simulink model "PIL_NO_RPI_new"  (R2021a)
settings: Solver=FixedStepAuto  StartTime=0.0  StopTime=60  FixedStep=0.001  RelTol=1e-3  EnableMultiTasking=on
values from neighbouring files (symbols this model uses):
  den_lpf_d = den_lpf20    [Mainframe_init.m]    (also in load_autopilot.m)
  Enable_Gyros = 0    [Mainframe_init.m]
  Enable_INS = 0    [Mainframe_init.m]
  num_lpf_d = num_lpf20    [Mainframe_init.m]    (also in load_autopilot.m)
undefined symbols (not defined in the file or in its folder): act_dmp, act_omega, Actuator, Aerodynamics, aMode, Autopilot, AUX, c_b_WGS, c_be, c_flat, c_grav, c_h_geop0, c_h_geope, c_pa0, c_pe, c_r0, c_rot, c_rsma, c_Tmp0, d_siB_0, d_siB_max, d_siB_min, dd_siB_max, dd_siB_min, dev, DiscIntNeverNeededParam, e_pa, e_Tmp, fin_maxrate, flag_I_act_switch, flag_I_aero_switch, flag_I_flat, flag_I_gravity_switch, flag_I_rot, h_bkpts_m, hcr, HIL_Data, JMMM_0, JMMM_e, JSPB_e, Ki_phi_vec, Kp_p_vec, Kp_phi_vec, lat_0, lon_0, Mass_Props, mB_0, mM_0, mM_e, National_Instruments, Newton, p, pBII_0, PCIe, phi, pMPB, pNPB, propellant_kg, prp_FBPB, prp_mdot ... (+40)
libraries: simulink x32, simulink_extras x23, aerolibcommonsys x4, pil_lib x2, custom_blocks x1, px4lib x1, sldrtlib x1, aerolibnav x1
(part 4 of 16)

== system PIL_NO_RPI_new/Non-linear Flight Dynamic Model1/GRM_Airframe/fin_actuators/Rudder3 ==
  siB_c : Inport
  tRRR : Inport  Port=2
  Add : Sum  Inputs=+-
  Add1 : Sum  Inputs=+-
  Add3 : Sum  Inputs=+++
  Constant1 : Constant  Value=Actuator.fin4_bias
      settings: AttributesFormatString=%<Value>
  Gain : Gain  Gain=omega^2
  Gain2 : Gain  Gain=2*dmp*omega  Multiplication=Matrix(K*u)
  Gain3 : Gain  Gain=unc_bl
  Gain4 : Gain  Gain=Actuator.fin4_scale
      settings: AttributesFormatString=%<Gain>
  Integrator : Integrator  ExternalReset=either  InitialCondition=d_siB_0
  Integrator1 : Integrator  InitialCondition=siB_0  LimitOutput=on  UpperSaturationLimit=siB_max  LowerSaturationLimit=siB_min  ShowSaturationPort=on
  Limiting_Acceleration : MATLAB Function  TreatAsAtomicUnit=on
  Limiting_Rate : MATLAB Function  TreatAsAtomicUnit=on
  Saturation : Saturate  UpperLimit=siB_max  LowerLimit=siB_min
  Saturation1 : Saturate  UpperLimit=siB_max  LowerLimit=siB_min
  Sign : Signum
  siB : Outport  VectorParamsAs1DForOutWhenUnconnected=off
  d_siB : Outport  Port=2  VectorParamsAs1DForOutWhenUnconnected=off
  dd_siB : Outport  Port=3  VectorParamsAs1DForOutWhenUnconnected=off
  wires:
  Saturation1/1 -> siB/1, [siB]  "siB"
  Integrator1/2 -> Integrator/2  "sat"
  Gain3/1 -> Add3/3
  Sign/1 -> Gain3/1
  tRRR/1 -> Sign/1  "tRRR"
  Integrator1/1 -> Gain4/1, Add/2  "siB"
  Add1/1 -> Limiting_Acceleration/3(dd_siB)  "dd_siB"
  Gain2/1 -> Add1/2
  Gain/1 -> Add1/1
  Add/1 -> Gain/1
  Limiting_Acceleration/1(dd_siB_l) -> Integrator/1, dd_siB/1  "dd_siB_l"
  Limiting_Rate/1(d_siB_l) -> d_siB/1, [d_siB], Integrator1/1  "d_siB_l"
  Integrator/1 -> Limiting_Rate/2(d_siB), Gain2/1  "d_siB"
  Saturation/1 -> Add/1
  Add3/1 -> Saturation1/1
  siB_c/1 -> Saturation/1  "siB_c"
  [d_siB] -> Limiting_Acceleration/2(d_siB)
  [siB] -> Limiting_Acceleration/1(siB)
  [siB] -> Limiting_Rate/1(siB)
  Constant1/1 -> Add3/1
  Gain4/1 -> Add3/2

== system PIL_NO_RPI_new/Non-linear Flight Dynamic Model1/GRM_Airframe/fin_actuators/control_allocation ==
  siB : Inport
  d_siB : Inport  Port=2
  dd_siB : Inport  Port=3
  Constant8 : Constant  Value=Tr3r4
  Product : Product  Multiplication=Matrix(*)
  Product1 : Product  Multiplication=Matrix(*)
  Product2 : Product  Multiplication=Matrix(*)
  Tr3r4 : Outport  VectorParamsAs1DForOutWhenUnconnected=off
  finB : Outport  Port=2  VectorParamsAs1DForOutWhenUnconnected=off
  d_finB : Outport  Port=3  VectorParamsAs1DForOutWhenUnconnected=off
  dd_finB : Outport  Port=4  VectorParamsAs1DForOutWhenUnconnected=off
  wires:
  Product/1 -> finB/1  "afinB"
  Constant8/1 -> Tr3r4/1, Product2/1, Product1/1, Product/1  "Tr3r4"
  siB/1 -> Product/2
  d_siB/1 -> Product1/2
  Product1/1 -> d_finB/1  "d_afinB"
  dd_siB/1 -> Product2/2
  Product2/1 -> dd_finB/1  "dd_afinB"

== system PIL_NO_RPI_new/Non-linear Flight Dynamic Model1/GRM_Airframe/gravity/launch_rail ==
  gBG_c : Inport
  hBE : Inport  Port=2
  Constant1 : Constant  Value=flag_I_gravity_switch
  Constant3 : Constant  Value=0
  Subtract : Sum  Inputs=++-
  Switch : Switch  Criteria=u2 > Threshold  Threshold=0.05
  Vector Concatenate : Concatenate  NumInputs=3
  initial_altitude : Subsystem
  gBG : Outport  VectorParamsAs1DForOutWhenUnconnected=off
  wires:
  Constant1/1 -> Subtract/2
  hBE/1 -> Subtract/1
  Subtract/1 -> Switch/2
  Constant3/1 -> Vector Concatenate/1, Vector Concatenate/2, Vector Concatenate/3
  Switch/1 -> gBG/1  "gBG"
  Vector Concatenate/1 -> Switch/3
  gBG_c/1 -> Switch/1
  initial_altitude/1(hBE_0) -> Subtract/3

== system PIL_NO_RPI_new/Non-linear Flight Dynamic Model1/GRM_Airframe/motion_kinematics/calc_motion_kinematics ==
  lat : Inport
  lon : Inport  Port=2
  qIB : Inport  Port=3
  calc_transformation_matrix : Subsystem
  earth_rotation : Subsystem
  wIEE : Outport  VectorParamsAs1DForOutWhenUnconnected=off
  TIE : Outport  Port=2  VectorParamsAs1DForOutWhenUnconnected=off
  TEB : Outport  Port=3  VectorParamsAs1DForOutWhenUnconnected=off
  TGB : Outport  Port=4  VectorParamsAs1DForOutWhenUnconnected=off
  TEG : Outport  Port=5  VectorParamsAs1DForOutWhenUnconnected=off
  wEGG : Outport  Port=6  VectorParamsAs1DForOutWhenUnconnected=off
  TIB : Outport  Port=7  VectorParamsAs1DForOutWhenUnconnected=off
  wires:
  earth_rotation/1(wIEE) -> wIEE/1
  earth_rotation/2(TIE) -> TIE/1
  earth_rotation/5(TEG) -> TEG/1
  earth_rotation/6(wEGG) -> wEGG/1
  lon/1 -> earth_rotation/2(lon)
  lat/1 -> earth_rotation/1(lat)
  earth_rotation/3(qIE) -> calc_transformation_matrix/1(qIE)
  earth_rotation/4(qEG) -> calc_transformation_matrix/2(qEG)
  qIB/1 -> calc_transformation_matrix/3(qIB)
  calc_transformation_matrix/1(TEB) -> TEB/1
  calc_transformation_matrix/2(TGB) -> TGB/1
  calc_transformation_matrix/3(TIB) -> TIB/1

== system PIL_NO_RPI_new/Non-linear Flight Dynamic Model1/GRM_Airframe/propulsion/prp_look_up ==
  env_glbl_bus : Inport
  Bus Selector1 : BusSelector  OutputSignals=T_sim_glbl,T_sim_lnch
  Constant : Constant  Value=0
  Constant1 : Constant  Value=0
  Saturation : Saturate  UpperLimit=prp_T(end)  LowerLimit=0
      settings: AttributesFormatString=|
      | %<UpperLimit>
      | %<LowerLimit>
  Subtract : Sum  Inputs=+-
  Switch : Switch  Criteria=u2 > Threshold
  Switch1 : Switch  Criteria=u2 > Threshold
  Vector Concatenate : Concatenate  NumInputs=3
  thrust_lookup : Lookup_n-D  NumberOfTableDimensions=1  BreakpointsForDimension1=prp_T  Table=prp_FBPB  ExtrapMethod=Clip  UseLastTableValue=on  InternalRulePriority=Speed  RndMeth=Simplest  InputSameDT=on
  FBPM : Outport  VectorParamsAs1DForOutWhenUnconnected=off
  wires:
  Bus Selector1/2 -> Subtract/2  "<T_sim_lnch>"
  Switch/1 -> Saturation/1, Switch1/2, Switch1/3
  thrust_lookup/1 -> Switch1/1
  Bus Selector1/1 -> Subtract/1  "<T_sim_glbl>"
  env_glbl_bus/1 -> Bus Selector1/1
  Constant/1 -> Switch/3
  Subtract/1 -> Switch/1, Switch/2
  Saturation/1 -> thrust_lookup/1
  Vector Concatenate/1 -> FBPM/1  "FBPM"
  Constant1/1 -> Vector Concatenate/3, Vector Concatenate/2
  Switch1/1 -> Vector Concatenate/1  "a_FBPM"

== system PIL_NO_RPI_new/Non-linear Flight Dynamic Model1/GRM_Airframe/propulsion/prp_uncertainty ==
  FBPM : Inport
  wab : Inport  Port=2
  3_rot_mat : Subsystem  mask(Rotation um 1, 2 oder 3 Achsen){rot_1=Rotation um z-Achse, rot_2=Rotation um y-Achse, rot_3=Rotation um x-Achse}
      mask prompts: rot_1 "1. Rotation"; rot_2 "2. Rotation"; rot_3 "3. Rotation"
      mask help:
      | Dieser Block liefert die Rotationsmatrix T12 für den Fall zurück, dass sich das Ziel-Koordinatensystem (1) durch Drehungen um 1, 2 oder 3 Achsen gegenüber dem Ausgangskoordinatensystem (2) beschreiben lässt (passive Drehung).
      |
      | Die Anzahl der Rotation sowie die Reihenfolge ist frei einstellbar.
      |
      | Die Rotationswinkel haben die Einheit [rad].
      mask TypeOptions rot_1: Rotation um x-Achse | Rotation um y-Achse | Rotation um z-Achse
      mask TypeOptions rot_2: Rotation um x-Achse | Rotation um y-Achse | Rotation um z-Achse
      mask TypeOptions rot_3: Rotation um x-Achse | Rotation um y-Achse | Rotation um z-Achse
  Bus Selector : BusSelector  OutputSignals=pBPB
  Product : Product  Multiplication=Matrix(*)
  Product1 : Product
  Subtract : Sum  Inputs=+-
  Thrust_rot_z : Constant  Value=unc_prp_z
  cross_product : Subsystem
      mask help: cross product r3 = r1 x r2
      mask Help:
      | Name:
      | 
      |     cross_product
      | 
      | Description:
      | 
      |     This block implements the cross product r3 = r1 x r2.
      | 
      | Inputs  [size] [data type] [unit]:
      | 
      |     vector 1  [3] [double] [-]
      |     vector 2  [3] [double] [-]
      | 
      | Outputs  [size] [data type] [unit]:
      | 
      |     resulting vector  [3] [double] [-]
      mask Display: disp(' r3 = r1 x r2')
  pNPB : Constant  Value=pNPB
  thrust_rot_x : Constant  Value=unc_prp_x
  thrust_rot_y : Constant  Value=unc_prp_y
  uncert_thrust : Constant  Value=unc_prp_scale
  FBPB : Outport  VectorParamsAs1DForOutWhenUnconnected=off
  MBPB : Outport  Port=2  VectorParamsAs1DForOutWhenUnconnected=off
  wires:
  Thrust_rot_z/1 -> 3_rot_mat/1(wi1)
  thrust_rot_x/1 -> 3_rot_mat/3(wi3)
  Product/1 -> cross_product/2(r2), FBPB/1  "FBPB"
  FBPM/1 -> Product1/1
  3_rot_mat/1(T12) -> Product/1
  thrust_rot_y/1 -> 3_rot_mat/2(wi2)
  cross_product/1(r1_x_r2) -> MBPB/1  "MBPB"
  wab/1 -> Bus Selector/1
  Bus Selector/1 -> Subtract/1  "<pBPB>"
  uncert_thrust/1 -> Product1/2
  Product1/1 -> Product/2
  pNPB/1 -> Subtract/2
  Subtract/1 -> cross_product/1(r1)

== system PIL_NO_RPI_new/Non-linear Flight Dynamic Model1/GRM_Airframe/rb_eom/calc_bus_flight_dyn_bus_entries ==
  mot_kin : Inport
  eom : Inport  Port=2
  Bus Selector : BusSelector  OutputSignals=pBII,vBII,qIB,wBIB,d_wBIB,d_vBII
  Bus Selector1 : BusSelector  OutputSignals=pBII
  Bus Selector3 : BusSelector  OutputSignals=TGB,TIB,TIE
  Constant : Constant  Value=pBII_0
      settings: AttributesFormatString=%<Value>
  Gain : Gain  Gain=-1
  Math Function : Math  Operator=transpose  SignedPower=on  SaturateOnIntegerOverflow=on
  Product{,1..3} (4 alike) : Product  Multiplication=Matrix(*)
  Subsystem2 : Subsystem
  Sum : Sum  Inputs=+-
  eom D1 : InportShadow  Port=2
  q12_from_T12 : Subsystem
      mask help: Transforms a Direction Cosine Matrix into a Quaternion
      mask Help:
      | Name:
      | 
      |     q12_from_T12
      | 
      | Description:
      | 
      |     This block implements the transformation of a direction cosine matrix DCM
      |      into the corresponding quaternion.
      | 
      | Inputs  [size] [data type] [unit]:
      | 
      |     direction cosine matrix T12  [3x3] [double] [-]
      | 
      | Outputs  [size] [data type] [unit]:
      | 
      |     quaternion q12  [4] [double] [-]
      mask Display:
      | %port_label('input', 1, 'T12')
      | %port_label('output', 1, 'q12')
      | disp('DCM \rightarrow q','texmode','on')
  quaternion_to_euler_angles : Subsystem
      mask help: transforms quaternions to Euler angles (roll, pitch, yaw)
      mask Help:
      | Name:
      | 
      |     quaternion_to_euler_angles
      | 
      | Description:
      | 
      |     This block implements the transformation of a quaternion into the
      |     corresponding Euler angles (zyx-sequence, roll, pitch, yaw).
      | 
      | Inputs  [size] [data type] [unit]:
      | 
      |     quaternion  [4] [double] [-]
      | 
      | Outputs  [size] [data type] [unit]:
      | 
      |     roll angle phi  [1] [double] [rad]
      |     pitch angle theta  [1] [double] [rad]
      |     yaw angle psi  [1] [double] [rad]
      mask Display:
      | %disp (' q --> (Phi,Theta,Psi) [rad]')
      | disp('q \rightarrow eu(\Phi;\Theta;\Psi)','texmode','on')
  quaternion_to_euler_angles1 : Subsystem
      mask help: transforms quaternions to Euler angles (roll, pitch, yaw)
      mask Help:
      | Name:
      | 
      |     quaternion_to_euler_angles
      | 
      | Description:
      | 
      |     This block implements the transformation of a quaternion into the
      |     corresponding Euler angles (zyx-sequence, roll, pitch, yaw).
      | 
      | Inputs  [size] [data type] [unit]:
      | 
      |     quaternion  [4] [double] [-]
      | 
      | Outputs  [size] [data type] [unit]:
      | 
      |     roll angle phi  [1] [double] [rad]
      |     pitch angle theta  [1] [double] [rad]
      |     yaw angle psi  [1] [double] [rad]
      mask Display:
      | %disp (' q --> (Phi,Theta,Psi) [rad]')
      | disp('q \rightarrow eu(\Phi;\Theta;\Psi)','texmode','on')
  aBIB : Outport  VectorParamsAs1DForOutWhenUnconnected=off
  lon : Outport  Port=2  VectorParamsAs1DForOutWhenUnconnected=off
  lat : Outport  Port=3  VectorParamsAs1DForOutWhenUnconnected=off
  hBE : Outport  Port=4  VectorParamsAs1DForOutWhenUnconnected=off
  vBII : Outport  Port=5  VectorParamsAs1DForOutWhenUnconnected=off
  qIB : Outport  Port=6  VectorParamsAs1DForOutWhenUnconnected=off
  wBIB : Outport  Port=7  VectorParamsAs1DForOutWhenUnconnected=off
  d_wBIB : Outport  Port=8  VectorParamsAs1DForOutWhenUnconnected=off
  d_vBII : Outport  Port=9  VectorParamsAs1DForOutWhenUnconnected=off
  pBII : Outport  Port=10  VectorParamsAs1DForOutWhenUnconnected=off
  euIB : Outport  Port=11  VectorParamsAs1DForOutWhenUnconnected=off
  vBIB : Outport  Port=12  VectorParamsAs1DForOutWhenUnconnected=off
  qGB : Outport  Port=13  VectorParamsAs1DForOutWhenUnconnected=off
  euGB : Outport  Port=14  VectorParamsAs1DForOutWhenUnconnected=off
  euBG : Outport  Port=15  VectorParamsAs1DForOutWhenUnconnected=off
  pBLG : Outport  Port=16  VectorParamsAs1DForOutWhenUnconnected=off
  wires:
  Bus Selector/1 -> pBII/1, Subsystem2/2(pBII)  "<pBII>"
  mot_kin/1 -> Bus Selector3/1
  Bus Selector3/3 -> Subsystem2/1(TIE)  "<TIE>"
  eom/1 -> Bus Selector/1
  Math Function/1 -> [TBI], Product1/1, Product/1  "TBI"
  Bus Selector3/2 -> Math Function/1  "<TIB>"
  Bus Selector/6 -> Product/2, d_vBII/1  "<d_vBII>"
  Product/1 -> aBIB/1  "aBIB"
  Subsystem2/1(lon) -> lon/1
  Subsystem2/2(lat) -> lat/1
  Subsystem2/3(hBE) -> hBE/1  "hBE"
  Bus Selector/2 -> Product1/2, vBII/1  "<vBII>"
  Bus Selector/3 -> quaternion_to_euler_angles/1(q), qIB/1  "<qIB>"
  Bus Selector/4 -> wBIB/1  "<wBIB>"
  Bus Selector/5 -> d_wBIB/1  "<d_wBIB>"
  quaternion_to_euler_angles/1(eulx) -> euIB/1  "euIB"
  Product1/1 -> vBIB/1  "vBIB"
  Bus Selector3/1 -> [TGB], q12_from_T12/1(T12)  "<TGB>"
  q12_from_T12/1(q12) -> quaternion_to_euler_angles1/1(q), qGB/1  "qGB"
  quaternion_to_euler_angles1/1(eulx) -> euGB/1, Gain/1  "euGB"
  Gain/1 -> euBG/1  "euBG"
  eom D1/1 -> Bus Selector1/1
  Bus Selector1/1 -> Sum/1  "<pBII>"
  Constant/1 -> Sum/2
  Sum/1 -> Product3/2  "pBLI"
  [TGB] -> Product2/1
  [TBI] -> Product2/2
  Product2/1 -> Product3/1  "TGI"
  Product3/1 -> pBLG/1  "pBLG"

== system PIL_NO_RPI_new/Non-linear Flight Dynamic Model1/GRM_Airframe/rb_eom/eom_6dof ==
  for_mom : Inport
  wab : Inport  Port=2
  Bus Selector1 : BusSelector  OutputSignals=mB,JBBB
  Bus Selector2 : BusSelector  OutputSignals=FBTB,MBTB
  Constant : Constant  Value=[pBII_0; vBII_0; qIB_0; wBIB_0]
  Constant9 : Constant  Value=[0 0 0; 0 0 0; 0 0 0]
  Rigid_Body_EOM_6_DOF : Subsystem  mask{flag_Kraft=FBTB}
      mask prompts: flag_Kraft "Input Kraftvektor"
      mask help:
      | 6DOF-Bewegungsgleichungen im ECI-System mit
      | zeitvariantem Massenträgheitsmoment.
      |
      | Modell Varianten:
      | - Koordinatensystem des Kraftvektor:
      |      FBTI : Inertial System I
      |      FBTB : Körperfestes System B
      mask init:
      | switch flag_Kraft
      |     case 1
      |         port_label_kraft = 'FBTI';
      |     case 2
      |         port_label_kraft = 'FBTB';
      | end
      mask TypeOptions flag_Kraft: FBTI | FBTB
      mask DialogControl Container4 Prompt: Modell Einstellungen
      mask Display:
      | port_label ('input',1,port_label_kraft )
      | port_label ('input',2,'MBTB' )
      | port_label ('input',3,'mB' )
      | port_label ('input',4,'x0' )
      | port_label ('input',5,'JBB' )
      | port_label ('input',6,'d_JBB' )
      | port_label ('output',1,'rb_eom' )
  eom : Outport  VectorParamsAs1DForOutWhenUnconnected=off
  wires:
  Bus Selector2/2 -> Rigid_Body_EOM_6_DOF/2(MBTB)  "<MBTB>"
  Bus Selector2/1 -> Rigid_Body_EOM_6_DOF/1(FBTX)  "<FBTB>"
  Rigid_Body_EOM_6_DOF/1(rb_eom) -> eom/1
  Constant9/1 -> Rigid_Body_EOM_6_DOF/6(d_JBB)
  Bus Selector1/2 -> Rigid_Body_EOM_6_DOF/5(JBB)  "<JBBB>"
  for_mom/1 -> Bus Selector2/1
  Constant/1 -> Rigid_Body_EOM_6_DOF/4(x0)
  Bus Selector1/1 -> Rigid_Body_EOM_6_DOF/3(mB)  "<mB>"
  wab/1 -> Bus Selector1/1

== system PIL_NO_RPI_new/Non-linear Flight Dynamic Model1/GRM_Airframe/stream_flow/calc_stream_flow ==
  TIB : Inport
  wIEE : Inport  Port=2
  TIE : Inport  Port=3
  VBII : Inport  Port=4
  pBII : Inport  Port=5
  wBIB : Inport  Port=6
  rho : Inport  Port=7
  sos : Inport  Port=8
  hBE : Inport  Port=9
  Bus Creator : BusCreator  Inputs=9
  Math Function : Math  Operator=transpose  SignedPower=on  SaturateOnIntegerOverflow=on
  Product : Product  Multiplication=Matrix(*)
  Subsystem1 : Subsystem
  velocity_vector_transformation : Subsystem
  str_flow : Outport  VectorParamsAs1DForOutWhenUnconnected=off
  wires:
  Subsystem1/4(MaB) -> Bus Creator/4
  Math Function/1 -> Product/1  "TBI"
  Subsystem1/2(be) -> Bus Creator/2  "beB"
  Subsystem1/8(fi) -> Bus Creator/8  "fiB"
  VBII/1 -> velocity_vector_transformation/3(vBII)
  Subsystem1/5(a_vB) -> Bus Creator/5
  Product/1 -> Subsystem1/1(vBEB)  "vBEB"
  Subsystem1/6(wBIB_star) -> Bus Creator/6
  TIE/1 -> velocity_vector_transformation/2(TIE)
  Subsystem1/3(qdynB) -> Bus Creator/3
  velocity_vector_transformation/1(vBEI) -> Product/2
  Subsystem1/7(th) -> Bus Creator/7  "inB"
  Subsystem1/1(al) -> Bus Creator/1  "alB"
  wIEE/1 -> velocity_vector_transformation/1(wIEE)
  Bus Creator/1 -> str_flow/1  "str_flow_bus"
  wBIB/1 -> Subsystem1/2(wBIB)
  hBE/1 -> Bus Creator/9
  sos/1 -> Subsystem1/4(sos)
  rho/1 -> Subsystem1/3(rho)
  TIB/1 -> Math Function/1
  pBII/1 -> velocity_vector_transformation/4(pBII)

== system PIL_NO_RPI_new/Non-linear Flight Dynamic Model1/GRM_Airframe/weight_and_balance/center_of_gravity ==
  mB : Inport
  mM : Inport  Port=2
  1-D Lookup Table : Lookup_n-D  NumberOfTableDimensions=1  BreakpointsForDimension1=Mass_Props.propellant_bkpts  Table=Mass_Props.CGx_m_tbl  ExtrapMethod=Clip  UseLastTableValue=on  InternalRulePriority=Speed  RndMeth=Simplest  InputSameDT=on
      settings: AttributesFormatString=|
      | %<Table>
      | %<BreakpointsForDimension1>
  1-D Lookup Table3 : Lookup_n-D  NumberOfTableDimensions=1  BreakpointsForDimension1=Mass_Props.propellant_bkpts  Table=Mass_Props.CGy_m_tbl  ExtrapMethod=Clip  UseLastTableValue=on  InternalRulePriority=Speed  RndMeth=Simplest  InputSameDT=on
      settings: AttributesFormatString=|
      | %<Table>
      | %<BreakpointsForDimension1>
  1-D Lookup Table6 : Lookup_n-D  NumberOfTableDimensions=1  BreakpointsForDimension1=Mass_Props.propellant_bkpts  Table=Mass_Props.CGz_m_tbl  ExtrapMethod=Clip  UseLastTableValue=on  InternalRulePriority=Speed  RndMeth=Simplest  InputSameDT=on
      settings: AttributesFormatString=|
      | %<Table>
      | %<BreakpointsForDimension1>
  Add6 : Sum
  Add7 : Sum
  Add8 : Sum
  Constant10 : Constant  Value=unc_cg_x
  Constant11 : Constant  Value=unc_cg_y
  Constant12 : Constant  Value=unc_cg_z
  Terminator1 : Terminator
  Vector Concatenate1 : Concatenate  NumInputs=3
  mM D2 : InportShadow  Port=2
  mM D3 : InportShadow  Port=2
  pBPB : Outport  VectorParamsAs1DForOutWhenUnconnected=off
  wires:
  1-D Lookup Table6/1 -> Add8/1
  1-D Lookup Table3/1 -> Add7/1
  Vector Concatenate1/1 -> pBPB/1  "pBPB"
  1-D Lookup Table/1 -> Add6/1
  mM/1 -> 1-D Lookup Table/1
  mM D2/1 -> 1-D Lookup Table3/1
  mM D3/1 -> 1-D Lookup Table6/1
  Add6/1 -> Vector Concatenate1/1
  Constant10/1 -> Add6/2
  Constant11/1 -> Add7/2
  Add7/1 -> Vector Concatenate1/2
  Constant12/1 -> Add8/2
  Add8/1 -> Vector Concatenate1/3
  mB/1 -> Terminator1/1

== system PIL_NO_RPI_new/Non-linear Flight Dynamic Model1/GRM_Airframe/weight_and_balance/mass ==
  sim_time_launch : Inport
  1-D Lookup Table2 : Lookup_n-D  NumberOfTableDimensions=1  BreakpointsForDimension1=prp_T  Table=prp_mdot  ExtrapMethod=Clip  DiagnosticForOutOfRangeInput=Warning  UseLastTableValue=on  InternalRulePriority=Speed  RndMeth=Simplest  InputSameDT=on
  Constant : Constant  Value=0
  Constant1 : Constant  Value=mB_0
  Constant2 : Constant  Value=propellant_kg
      settings: AttributesFormatString=%<Value>
  Gain : Gain  Gain=-1
  Integrator1 : Integrator  InitialConditionSource=external
  Saturation : Saturate  UpperLimit=prp_T(end)  LowerLimit=0
      settings: AttributesFormatString=|
      | %<UpperLimit>
      | %<LowerLimit>
  Subtract1 : Sum
  Switch : Switch  Criteria=u2 > Threshold
  Switch1 : Switch  Criteria=u2 > Threshold
  mB_c : Outport  VectorParamsAs1DForOutWhenUnconnected=off
  mM : Outport  Port=2  VectorParamsAs1DForOutWhenUnconnected=off
  wires:
  Constant1/1 -> Subtract1/1
  Subtract1/1 -> mB_c/1  "mB_c"
  Switch/1 -> Switch1/2, Switch1/3, Saturation/1
  Constant/1 -> Switch/3
  sim_time_launch/1 -> Switch/1, Switch/2
  Saturation/1 -> 1-D Lookup Table2/1
  Switch1/1 -> mM/1, Subtract1/2  "mM"
  Constant2/1 -> Integrator1/2
  1-D Lookup Table2/1 -> Gain/1  "mdot_kgps"
  Gain/1 -> Integrator1/1
  Integrator1/1 -> Switch1/1  "propellant_remaining_kg"

== system PIL_NO_RPI_new/Non-linear Flight Dynamic Model1/GRM_Airframe/weight_and_balance/mass_uncertainty ==
  mB_c : Inport
  Add : Sum
  Constant : Constant  Value=unc_mB_bl
  Constant1 : Constant  Value=unc_mB_scale
  Product : Product
  mB : Outport  VectorParamsAs1DForOutWhenUnconnected=off
  wires:
  Constant/1 -> Add/1
  mB_c/1 -> Product/1
  Add/1 -> mB/1  "mB"
  Constant1/1 -> Product/2
  Product/1 -> Add/2

== system PIL_NO_RPI_new/Non-linear Flight Dynamic Model1/GRM_Airframe/weight_and_balance/moi ==
  pBPB : Inport
  mM : Inport  Port=2
  1-D Lookup Table : Lookup_n-D  NumberOfTableDimensions=1  BreakpointsForDimension1=Mass_Props.propellant_bkpts  Table=Mass_Props.Ixx_tbl  ExtrapMethod=Clip  UseLastTableValue=on  InternalRulePriority=Speed  RndMeth=Simplest  InputSameDT=on
      settings: AttributesFormatString=|
      | %<Table>
      | %<BreakpointsForDimension1>
  1-D Lookup Table1 : Lookup_n-D  NumberOfTableDimensions=1  BreakpointsForDimension1=Mass_Props.propellant_bkpts  Table=Mass_Props.Ixy_tbl  ExtrapMethod=Clip  UseLastTableValue=on  InternalRulePriority=Speed  RndMeth=Simplest  InputSameDT=on
      settings: AttributesFormatString=|
      | %<Table>
      | %<BreakpointsForDimension1>
  1-D Lookup Table2 : Lookup_n-D  NumberOfTableDimensions=1  BreakpointsForDimension1=Mass_Props.propellant_bkpts  Table=Mass_Props.Ixz_tbl  ExtrapMethod=Clip  UseLastTableValue=on  InternalRulePriority=Speed  RndMeth=Simplest  InputSameDT=on
      settings: AttributesFormatString=|
      | %<Table>
      | %<BreakpointsForDimension1>
  1-D Lookup Table3 : Lookup_n-D  NumberOfTableDimensions=1  BreakpointsForDimension1=Mass_Props.propellant_bkpts  Table=Mass_Props.Iyx_tbl  ExtrapMethod=Clip  UseLastTableValue=on  InternalRulePriority=Speed  RndMeth=Simplest  InputSameDT=on
      settings: AttributesFormatString=|
      | %<Table>
      | %<BreakpointsForDimension1>
  1-D Lookup Table4 : Lookup_n-D  NumberOfTableDimensions=1  BreakpointsForDimension1=Mass_Props.propellant_bkpts  Table=Mass_Props.Iyy_tbl  ExtrapMethod=Clip  UseLastTableValue=on  InternalRulePriority=Speed  RndMeth=Simplest  InputSameDT=on
      settings: AttributesFormatString=|
      | %<Table>
      | %<BreakpointsForDimension1>
  1-D Lookup Table5 : Lookup_n-D  NumberOfTableDimensions=1  BreakpointsForDimension1=Mass_Props.propellant_bkpts  Table=Mass_Props.Iyz_tbl  ExtrapMethod=Clip  UseLastTableValue=on  InternalRulePriority=Speed  RndMeth=Simplest  InputSameDT=on
      settings: AttributesFormatString=|
      | %<Table>
      | %<BreakpointsForDimension1>
  1-D Lookup Table6 : Lookup_n-D  NumberOfTableDimensions=1  BreakpointsForDimension1=Mass_Props.propellant_bkpts  Table=Mass_Props.Izx_tbl  ExtrapMethod=Clip  UseLastTableValue=on  InternalRulePriority=Speed  RndMeth=Simplest  InputSameDT=on
      settings: AttributesFormatString=|
      | %<Table>
      | %<BreakpointsForDimension1>
  1-D Lookup Table7 : Lookup_n-D  NumberOfTableDimensions=1  BreakpointsForDimension1=Mass_Props.propellant_bkpts  Table=Mass_Props.Izy_tbl  ExtrapMethod=Clip  UseLastTableValue=on  InternalRulePriority=Speed  RndMeth=Simplest  InputSameDT=on
      settings: AttributesFormatString=|
      | %<Table>
      | %<BreakpointsForDimension1>
  1-D Lookup Table8 : Lookup_n-D  NumberOfTableDimensions=1  BreakpointsForDimension1=Mass_Props.propellant_bkpts  Table=Mass_Props.Izz_tbl  ExtrapMethod=Clip  UseLastTableValue=on  InternalRulePriority=Speed  RndMeth=Simplest  InputSameDT=on
      settings: AttributesFormatString=|
      | %<Table>
      | %<BreakpointsForDimension1>
  Add : Sum  Commented=on
  Add4 : Sum  Commented=on
  Add5 : Sum  Commented=on
  Constant15 : Constant  Commented=on  Value=JSPB_e
  JMMM_linear_interpolation : Subsystem  Commented=on
  Matrix Concatenate : Concatenate  NumInputs=3  Mode=Multidimensional array  ConcatenateDimension=2
  Terminator : Terminator  Commented=on
  Vector Concatenate : Concatenate  NumInputs=3
  Vector Concatenate1 : Concatenate  NumInputs=3
  Vector Concatenate2 : Concatenate  NumInputs=3
  mM D{1..9} (9 alike) : InportShadow  Port=2
  moi_coordinate_transformation : Subsystem  Commented=on
  moi_uncertainty : Subsystem
  steiners_theorem_missile : Subsystem  Commented=on
  steiners_theorem_motor : Subsystem  Commented=on
  JBBB : Outport  VectorParamsAs1DForOutWhenUnconnected=off
  wires:
  mM/1 -> steiners_theorem_motor/2(mM), JMMM_linear_interpolation/1(mM)
  JMMM_linear_interpolation/1(JMMM) -> moi_coordinate_transformation/1(JMMM)
  moi_coordinate_transformation/1(JMMB) -> Add/2
  pBPB/1 -> steiners_theorem_missile/1(pBPB), steiners_theorem_motor/1(pBPB)
  steiners_theorem_motor/1(JM_deviation) -> Add/1
  Add/1 -> Add4/2  "JMBB"
  Constant15/1 -> Add5/1
  Add5/1 -> Add4/1  "JSBB"
  steiners_theorem_missile/1(J_deviation) -> Add5/2
  Add4/1 -> Terminator/1  "JBBB_c"
  moi_uncertainty/1(JBBB) -> JBBB/1
  mM D1/1 -> 1-D Lookup Table/1
  mM D2/1 -> 1-D Lookup Table3/1
  mM D3/1 -> 1-D Lookup Table6/1
  mM D4/1 -> 1-D Lookup Table1/1
  mM D5/1 -> 1-D Lookup Table4/1
  mM D6/1 -> 1-D Lookup Table7/1
  mM D7/1 -> 1-D Lookup Table2/1
  mM D8/1 -> 1-D Lookup Table5/1
  mM D9/1 -> 1-D Lookup Table8/1
  1-D Lookup Table6/1 -> Vector Concatenate/3
  1-D Lookup Table3/1 -> Vector Concatenate/2
  1-D Lookup Table/1 -> Vector Concatenate/1
  1-D Lookup Table1/1 -> Vector Concatenate1/1
  1-D Lookup Table4/1 -> Vector Concatenate1/2
  1-D Lookup Table7/1 -> Vector Concatenate1/3
  1-D Lookup Table2/1 -> Vector Concatenate2/1
  1-D Lookup Table5/1 -> Vector Concatenate2/2
  1-D Lookup Table8/1 -> Vector Concatenate2/3
  Vector Concatenate/1 -> [MOI_matrix_col1]
  Vector Concatenate1/1 -> [MOI_matrix_col2]
  Vector Concatenate2/1 -> [MOI_matrix_col3]
  [MOI_matrix_col1] -> Matrix Concatenate/1
  [MOI_matrix_col2] -> Matrix Concatenate/2
  [MOI_matrix_col3] -> Matrix Concatenate/3
  Matrix Concatenate/1 -> moi_uncertainty/1(JBBB_c)  "JBBB_c"

== system PIL_NO_RPI_new/Non-linear Flight Dynamic Model1/Subsystem1/Extract States/Assemble_States_Bus1 ==
  Translation_States : Inport
  Rotation_States : Inport  Port=2
  Translation_States_Dot : Inport  Port=3
  Rotation_States_Dot : Inport  Port=4
  Attitude_States : Inport  Port=5
  POS_NED : Inport  Port=6
  POS_NED_dot : Inport  Port=7
  Bus Creator{1,4..6,8,12..13} (7 alike) : BusCreator  Inputs=3
  Bus Creator3 : BusCreator  Inputs=7
  Bus Creator7 : BusCreator  Inputs=2
  Bus Creator9 : BusCreator  Inputs=4
  Demux : Demux
  Demux{1..7} (7 alike) : Demux  Outputs=3
  Rotation Angles to Quaternions : Subsystem  mask(Ang2Quat){rotationOrder=ZYX, aMode=aMode}
      mask prompts: rotationOrder "shared_aeroblks:sharedaeroblktransform:blockAng2QuatParamRotationOrder"
      mask help: shared_aeroblks:sharedaeroblktransform:blockAng2QuatDesc
      mask init:
      | if aerosharedtest(gcb)
      |     ports=aerosharedicon('sharedang2quat');
      | else
      |     ports=sharedautoicon('sharedang2quat');
      | end
      settings: AttributesFormatString=Rotation Order: %<rotationOrder>
      mask Help: eval('if license(''test'',''Aerospace_Blockset'')aerosharedhelp(''rotation_angles_to_quaternions'');elseif license(''test'',''Powertrain_Blockset'')sharedautohelp(''rotation_angles_to_quaternions'');end')
      mask TypeOptions rotationOrder: shared_aeroblks:sharedaeroblktransform:blockParamComboZYX | shared_aeroblks:sharedaeroblktransform:blockParamComboZYZ | shared_aeroblks:sharedaeroblktransform:blockParamComboZXY | shared_aeroblks:sharedaeroblktransform:blockParamComboZXZ | shared_aeroblks:sharedaeroblktransform:blockParamComboYXZ | shared_aeroblks:sharedaeroblktransform:blockParamComboYXY | shared_aeroblks:sharedaeroblktransform:blockParamComboYZX | shared_aeroblks:sharedaeroblktransform:blockParamComboYZY | shared_aeroblks:sharedaeroblktransform:blockParamComboXYZ | shared_aeroblks:sharedaeroblktransform:blockParamComboXYX | shared_aeroblks:sharedaeroblktransform:blockParamComboXZY | shared_aeroblks:sharedaeroblktransform:blockParamComboXZX
      mask DialogControl rotationOrder Prompt: Rotation order:
      mask Display:
      | port_label('input',1,'[R_1,R_2,R_3]','texmode','on')
      | port_label('output',1,'q','texmode','on')
  Selector : Selector  InputPortWidth=3  IndexOptions=Index vector (dialog)  Indices=[3,2,1]  OutputSizes=1
  Three-axis Inertial Measurement Unit3 : Subsystem  Commented=on  mask(Three-axis Inertial Measurement Unit){units=Metric (MKS), imu=[0 0 0], i_Ts=0, dtype_a=on, w_a=190, z_a=0.707, a_sf_cc=[1 0 0; 0 1 0; 0 0 1], a_bias=[0 0 0], a_sat=[-inf  -inf  -inf  inf inf inf], dtype_g=on, w_g=190, z_g=0.707, g_sf_cc=[1 0 0; 0 1 0; 0 0 1], g_bias=[0 0 0], g_sens=[0 0 0], g_sat=[-inf  -inf  -inf  inf inf inf], i_rand=on, i_seeds=[23093 23094 23095 23096 23097 23098], i_pow=[0.001 0.001 0.001 0.0001 0.0001 0.0001]}
      mask prompts: units "aeroblks:aeroblknav:blockThreeaxisInertialMeasurementUnitParamUnits"; imu "aeroblks:aeroblknav:blockThreeaxisInertialMeasurementUnitParamIMUlocation"; i_Ts "aeroblks:aeroblknav:blockThreeaxisInertialMeasurementUnitParamUpdaterate"; dtype_a "aeroblks:aeroblknav:blockThreeaxisInertialMeasurementUnitParamSecondorderdynamicsforaccelerometer"; w_a "aeroblks:aeroblknav:blockThreeaxisInertialMeasurementUnitParamAccelerometernaturalfrequencyradsec"; z_a "aeroblks:aeroblknav:blockThreeaxisInertialMeasurementUnitParamAccelerometerdampingratio"; a_sf_cc "aeroblks:aeroblknav:blockThreeaxisInertialMeasurementUnitParamAccelerometerscalefactorandcrosscoupling"; a_bias "aeroblks:aeroblknav:blockThreeaxisInertialMeasurementUnitParamAccelerometermeasurementbias"; a_sat "aeroblks:aeroblknav:blockThreeaxisInertialMeasurementUnitParamAccelerometerupperandlowerlimits"; dtype_g "aeroblks:aeroblknav:blockThreeaxisInertialMeasurementUnitParamSecondorderdynamicsforgyro"; w_g "aeroblks:aeroblknav:blockThreeaxisInertialMeasurementUnitParamGyronaturalfrequencyradsec"; z_g "aeroblks:aeroblknav:blockThreeaxisInertialMeasurementUnitParamGyrodampingratio"; g_sf_cc "aeroblks:aeroblknav:blockThreeaxisInertialMeasurementUnitParamGyroscalefactorsandcrosscoupling"; g_bias "aeroblks:aeroblknav:blockThreeaxisInertialMeasurementUnitParamGyromeasurementbias"; g_sens "aeroblks:aeroblknav:blockThreeaxisInertialMeasurementUnitParamGsensitivebias"; g_sat "aeroblks:aeroblknav:blockThreeaxisInertialMeasurementUnitParamGyroupperandlowerlimits"; i_rand "aeroblks:aeroblknav:blockThreeaxisInertialMeasurementUnitParamNoiseon"; i_seeds "aeroblks:aeroblknav:blockThreeaxisInertialMeasurementUnitParamNoiseseeds"; i_pow "aeroblks:aeroblknav:blockThreeaxisInertialMeasurementUnitParamNoisepower"
      mask help: aeroblks:aeroblknav:blockThreeaxisInertialMeasurementUnitDesc
      mask init:
      | block = gcb;   
      | ports=aeroicon('aeroblkimu','icon');
      mask Help: eval('asbhelp');
      mask TypeOptions units: aeroblks:aeroblknav:blockThreeaxisInertialMeasurementUnitParamComboMetricMKS | aeroblks:aeroblknav:blockThreeaxisInertialMeasurementUnitParamComboEnglish
      mask Callback dtype_a: aeroicon('aeroblkimu')
      mask Callback dtype_g: aeroicon('aeroblkimu')
      mask Callback i_rand: aeroicon('aeroblkimu')
      mask DialogControl ParameterTabVar0 Prompt: Main
      mask DialogControl units Prompt: Units:
      mask DialogControl imu Prompt: IMU location:
      mask DialogControl i_Ts Prompt: Update rate:
      mask DialogControl ParameterTabVar01 Prompt: Accelerometer
      mask DialogControl dtype_a Prompt: Second-order dynamics for accelerometer
      mask DialogControl w_a Prompt: Accelerometer natural frequency (rad/sec):
      mask DialogControl z_a Prompt: Accelerometer damping ratio:
      mask DialogControl a_sf_cc Prompt: Accelerometer scale factor and cross-coupling:
      mask DialogControl a_bias Prompt: Accelerometer measurement bias:
      mask DialogControl a_sat Prompt: Accelerometer upper and lower limits:
      mask DialogControl ParameterTabVar012 Prompt: Gyroscope
      mask DialogControl dtype_g Prompt: Second-order dynamics for gyro
      mask DialogControl w_g Prompt: Gyro natural frequency (rad/sec):
      mask DialogControl z_g Prompt: Gyro damping ratio:
      mask DialogControl g_sf_cc Prompt: Gyro scale factors and cross-coupling:
      mask DialogControl g_bias Prompt: Gyro measurement bias:
      mask DialogControl g_sens Prompt: G-sensitive bias:
      mask DialogControl g_sat Prompt: Gyro upper and lower limits:
      mask DialogControl ParameterTabVar0123 Prompt: Noise
      mask DialogControl i_rand Prompt: Noise on
      mask DialogControl i_seeds Prompt: Noise seeds:
      mask DialogControl i_pow Prompt: Noise power:
      mask Display:
      | port_label(ports(1).type,ports(1).port,ports(1).txt,'texmode','on');
      | port_label(ports(2).type,ports(2).port,ports(2).txt,'texmode','on');
      | port_label(ports(3).type,ports(3).port,ports(3).txt,'texmode','on');
      | port_label(ports(4).type,ports(4).port,ports(4).txt,'texmode','on');
      | port_label(ports(5).type,ports(5).port,ports(5).txt,'texmode','on');
      | port_label(ports(6).type,ports(6).port,ports(6).txt,'texmode','on');
      | port_label(ports(7).type,ports(7).port,ports(7).txt,'texmode','on');
  States : Outport  VectorParamsAs1DForOutWhenUnconnected=off
  wires:
  Bus Creator7/1 -> Bus Creator3/5  "Attitude_States"
  Demux/3 -> Bus Creator9/3  "quat_2"
  Demux/4 -> Bus Creator9/4  "quat_3"
  Demux/1 -> Bus Creator9/1  "quat_0"
  Bus Creator9/1 -> Bus Creator7/2  "ATT_Quaternions"
  Bus Creator12/1 -> Bus Creator3/6  "POS_NED"
  Demux/2 -> Bus Creator9/2  "quat_1"
  Bus Creator8/1 -> Bus Creator7/1  "ATT_Euler"
  Bus Creator4/1 -> Bus Creator3/1  "Translation_States"
  Bus Creator6/1 -> Bus Creator3/2  "Rotation_States"
  Bus Creator5/1 -> Bus Creator3/3  "Translation_States_Dot"
  Rotation Angles to Quaternions/1(Quat) -> Demux/1
  Demux6/3 -> Bus Creator12/3  "POS_z_NED_m"
  Demux6/2 -> Bus Creator12/2  "POS_y_NED_m"
  Demux6/1 -> Bus Creator12/1  "POS_x_NED_m"
  Demux5/3 -> Bus Creator8/3  "Psi_rad"
  Demux5/2 -> Bus Creator8/2  "Theta_rad"
  Demux5/1 -> Bus Creator8/1  "Phi_rad"
  Demux2/3 -> Bus Creator6/3  "r_radDs"
  Demux2/2 -> Bus Creator6/2  "q_radDs"
  Demux2/1 -> Bus Creator6/1  "p_radDs"
  Demux3/3 -> Bus Creator5/3  "w_dot_mDs2"
  Demux3/2 -> Bus Creator5/2  "v_dot_mDs2"
  Demux3/1 -> Bus Creator5/1  "u_dot_mDs2"
  Demux1/3 -> Bus Creator4/3  "w_mDs"
  Demux1/2 -> Bus Creator4/2  "v_mDs"
  Demux1/1 -> Bus Creator4/1  "u_mDs"
  Bus Creator13/1 -> Bus Creator3/4  "Rotation_States_Dot"
  Demux4/1 -> Bus Creator13/1  "p_dot_radDs2"
  Demux4/2 -> Bus Creator13/2  "q_dot_radDs2"
  Demux4/3 -> Bus Creator13/3  "r_dot_radDs2"
  Translation_States/1 -> Demux1/1
  Rotation_States/1 -> Demux2/1
  Translation_States_Dot/1 -> Demux3/1
  Rotation_States_Dot/1 -> Demux4/1
  Attitude_States/1 -> Selector/1, Demux5/1
  POS_NED/1 -> Demux6/1
  Bus Creator3/1 -> States/1  "FDM_States"
  Selector/1 -> Rotation Angles to Quaternions/1("R1, R2, R3")
  POS_NED_dot/1 -> Demux7/1
  Demux7/2 -> Bus Creator1/2  "POS_y_NED_dot_m"
  Demux7/3 -> Bus Creator1/3  "POS_z_NED_dot_m"
  Bus Creator1/1 -> Bus Creator3/7  "POS_NED_dot"
  Demux7/1 -> Bus Creator1/1  "POS_x_NED_dot_m"

== system PIL_NO_RPI_new/Non-linear Flight Dynamic Model1/Subsystem1/Extract States/quaternion_to_euler_angles1 ==
  note: Um numerische Probleme zu
      | vermeiden, wird hier eine Saturiierung
      | benutzt.
  note: Outputs [size]:
      |
      | roll angle [1]
      | pitch angle [1]
      | yaw angle [1]
  note: Inputs [size]:
      |
      | quaternion [4]
  q : Inport  PortDimensions=4
  Add : Sum
  Add1 : Sum  Inputs=+--
  Add2 : Sum  Inputs=+-
  Add3 : Sum
  Add4 : Sum  Inputs=+--
  Complex to Real-Imag : ComplexToRealImag  Output=Real
  Constant : Constant  Value=0.5
  Constant1 : Constant  Value=0.5
  Demux : Demux
  Gain : Gain  Gain=2
  Product{,1..9} (10 alike) : Product
  Saturation : Saturate  UpperLimit=1  LowerLimit=-1
      settings: AttributesFormatString=|
      | %<UpperLimit>
      | %<LowerLimit>
  Trigonometric Function : Trigonometry  Operator=atan2
  Trigonometric Function1 : Trigonometry  Operator=asin
  Trigonometric Function2 : Trigonometry  Operator=atan2
  Vector Concatenate : Concatenate  NumInputs=3
  eulx : Outport  VectorParamsAs1DForOutWhenUnconnected=off
  wires:
  Vector Concatenate/1 -> Complex to Real-Imag/1
  Complex to Real-Imag/1 -> eulx/1
  Trigonometric Function2/1 -> Vector Concatenate/3
  Trigonometric Function1/1 -> Vector Concatenate/2
  Trigonometric Function/1 -> Vector Concatenate/1
  Add/1 -> Trigonometric Function/1
  Product1/1 -> Add/2
  Product/1 -> Add/1
  Product3/1 -> Add1/3
  Product2/1 -> Add1/2
  Product5/1 -> Add2/2
  Product4/1 -> Add2/1
  Product7/1 -> Add3/2
  Product6/1 -> Add3/1
  Add3/1 -> Trigonometric Function2/1
  Add4/1 -> Trigonometric Function2/2
  Add2/1 -> Gain/1
  Add1/1 -> Trigonometric Function/2
  q/1 -> Demux/1
  Demux/4 -> Product7/2, Product4/2, Product/2  "4"
  Demux/1 -> Product2/2, Product2/1, Product/1, Product6/1, Product5/1  "1"
  Demux/2 -> Product4/1, Product3/2, Product3/1, Product1/1, Product8/2, Product8/1, Product6/2  "2"
  Constant/1 -> Add1/1
  Product9/1 -> Add4/3
  Product8/1 -> Add4/2
  Constant1/1 -> Add4/1
  Demux/3 -> Product9/2, Product9/1, Product7/1, Product1/2, Product5/2  "3"
  Gain/1 -> Saturation/1
  Saturation/1 -> Trigonometric Function1/1

== system PIL_NO_RPI_new/Non-linear Flight Dynamic Model1/Subsystem1/Fin Deflections/Degrees to Radians ==
  Degrees in : Inport
  Gain1 : Gain  Gain=pi/180  SaturateOnIntegerOverflow=on  OutDataTypeStr=Inherit: Same as input  ParamDataTypeStr=Inherit: Same as input
  Radians out : Outport  InitialOutput=0  VectorParamsAs1DForOutWhenUnconnected=off
  wires:
  Gain1/1 -> Radians out/1
  Degrees in/1 -> Gain1/1

== system PIL_NO_RPI_new/Non-linear Flight Dynamic Model1/Subsystem1/Fin Deflections/Degrees to Radians1 ==
  Degrees in : Inport
  Gain1 : Gain  Gain=pi/180  SaturateOnIntegerOverflow=on  OutDataTypeStr=Inherit: Same as input  ParamDataTypeStr=Inherit: Same as input
  Radians out : Outport  InitialOutput=0  VectorParamsAs1DForOutWhenUnconnected=off
  wires:
  Gain1/1 -> Radians out/1
  Degrees in/1 -> Gain1/1

== system PIL_NO_RPI_new/Non-linear Flight Dynamic Model1/Subsystem1/Fin Deflections/Degrees to Radians2 ==
  Degrees in : Inport
  Gain1 : Gain  Gain=pi/180  SaturateOnIntegerOverflow=on  OutDataTypeStr=Inherit: Same as input  ParamDataTypeStr=Inherit: Same as input
  Radians out : Outport  InitialOutput=0  VectorParamsAs1DForOutWhenUnconnected=off
  wires:
  Gain1/1 -> Radians out/1
  Degrees in/1 -> Gain1/1

== system PIL_NO_RPI_new/Non-linear Flight Dynamic Model1/Subsystem1/Fin Deflections/control_allocation ==
  fin_cmd : Inport
  Constant7 : Constant  Value=Tr4r3
  Product : Product  Multiplication=Matrix(*)
  siB_cmd : Outport  VectorParamsAs1DForOutWhenUnconnected=off
  wires:
  Product/1 -> siB_cmd/1  "siB_cmd"
  fin_cmd/1 -> Product/2
  Constant7/1 -> Product/1

== system PIL_NO_RPI_new/Non-linear Flight Dynamic Model1/Subsystem1/GRM_Airframe/aerodynamics ==
  str_flow : Inport
  fin : Inport  Port=2
  wab : Inport  Port=3
  env_glbl : Inport  Port=4
  Bus Selector : BusSelector  OutputSignals=qdynB,MaB,alB,beB,hBE,wBIB_star
  Bus Selector1 : BusSelector  OutputSignals=afinB
  Bus Selector2 : BusSelector  OutputSignals=pBPB
  aerodynamic_via_lookup : Subsystem
  logic_base_drag : Subsystem
  aero : Outport  VectorParamsAs1DForOutWhenUnconnected=off
  wires:
  str_flow/1 -> Bus Selector/1
  wab/1 -> Bus Selector2/1
  fin/1 -> Bus Selector1/1
  Bus Selector2/1 -> aerodynamic_via_lookup/1(pBPB)  "<pBPB>"
  Bus Selector/1 -> aerodynamic_via_lookup/2(qdynB)  "<qdynB>"
  Bus Selector/2 -> aerodynamic_via_lookup/3(MaB)  "<MaB>"
  Bus Selector/3 -> aerodynamic_via_lookup/4(alB)  "<alB>"
  Bus Selector/4 -> aerodynamic_via_lookup/5(beB)  "<beB>"
  Bus Selector/5 -> aerodynamic_via_lookup/6(hBE)  "<hBE>"
  Bus Selector1/1 -> aerodynamic_via_lookup/8(afinB)  "<afinB>"
  Bus Selector/6 -> aerodynamic_via_lookup/7(wBIB_star)  "<wBIB_star>"
  aerodynamic_via_lookup/1(aero_bus) -> aero/1
  env_glbl/1 -> logic_base_drag/1(env_glbl)
  logic_base_drag/1(flag_base_drag) -> aerodynamic_via_lookup/9(flag_I_prp)

== system PIL_NO_RPI_new/Non-linear Flight Dynamic Model1/Subsystem1/GRM_Airframe/environment ==
  flight_dyn : Inport
  env_glbl : Inport  Port=2
  Bus Creator1 : BusCreator  Inputs=2
  Bus Creator2 : BusCreator  Inputs=2
  Bus Selector : BusSelector  OutputSignals=lon,lat,hBE
  Bus Selector1 : BusSelector  OutputSignals=atm_dyn_bus
  Saturation : Saturate  UpperLimit=inf  LowerLimit=eps
      settings: AttributesFormatString=|
      | %<UpperLimit>
      | %<LowerLimit>
  WGS84_Gravitation : Subsystem  mask{flg_omega_enabled=on}
      mask prompts: flg_omega_enabled "Zentripetalbeschleunigung mitberechnen"
      mask help:
      | Dieser Block berechnet die Gravitation für das idealisierte WGS84
      | Ellipsoid. Die Berechnung ist hierbei nach dem Technical Report
      | "Department of Defense World Geodetic System 1984", NIMA TR8350.2,
      | Third Edition, Amendment 1 vom 3 Januar 2000 implementiert.
      | Das Modell ist gültig für alle Höhen über dem WGS84 Referenzellipsoid, und
      | ist somit der reinen Taylorexpansion des Somigliana Modells überlegen
      | (siehe Kapitel 4.3 des WGS84 reports).
      |
      | ---------------------------------------------------------------------------
      | Longitude [rad]: Nach WGS84 definierte Geodätische Länge.  (lambda)
      | Lattitude [rad]: Nach WGS84 definierte Geodätische Breite. (phi)
      | Height [m]: Höhe über dem WGS84 Referenzellipsoid.
      mask init:
      | [ c_rsma, c_b_WGS, c_grav, c_rot] = init_WGS84_Gravitationsmodell();
  atmosphere_static_ISO_2533 : Subsystem
  convert_to_local_frame : Subsystem
  env : Outport  VectorParamsAs1DForOutWhenUnconnected=off
  wires:
  convert_to_local_frame/1(gBG) -> Bus Creator2/1
  flight_dyn/1 -> Bus Selector/1
  WGS84_Gravitation/1(gE) -> convert_to_local_frame/1(gE)
  Bus Selector/1 -> WGS84_Gravitation/1(lon)  "<lon>"
  Bus Selector/3 -> atmosphere_static_ISO_2533/1(hBE), Saturation/1  "<hBE>"
  Bus Creator2/1 -> env/1  "env_bus"
  Bus Selector/2 -> WGS84_Gravitation/2(lat)  "<lat>"
  Bus Creator1/1 -> Bus Creator2/2  "atm_bus"
  Saturation/1 -> WGS84_Gravitation/3(h)
  atmosphere_static_ISO_2533/1(atm_stat) -> Bus Creator1/1  "atm_stat_bus"
  env_glbl/1 -> Bus Selector1/1, atmosphere_static_ISO_2533/2(env_glbl)
  Bus Selector1/1 -> Bus Creator1/2  "<atm_dyn_bus>"
